simulink model "AmplitudeModulation"  (Simulink 7.5)
settings: Solver=ode45  StartTime=0.0  StopTime=5  RelTol=1e-3
settings Model: Creator=Terje B  LastModifiedBy=Terje B
settings DebuggingCC: SolverPrmCheckMsg=none

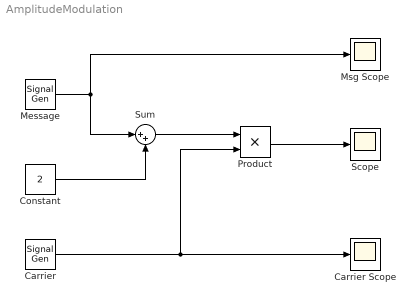
== system AmplitudeModulation ==
  Carrier : SignalGenerator  Frequency=10
  Carrier Scope : Scope
      settings: SaveName=ScopeData2
  Constant : Constant  Value=2  OutDataType=fixdt(1, 16)  OutScaling=2^0
  Message : SignalGenerator
  Msg Scope : Scope
  Product : Product  OutDataType=fixdt(1, 16)  OutScaling=2^0  SampleTime=.001  RndMeth=Zero
  Scope : Scope
  Sum : Sum  Inputs=|++  OutDataType=fixdt(1, 16)  OutScaling=2^0
  wires:
  Message/1 -> Sum/1, Msg Scope/1
  Constant/1 -> Sum/2
  Sum/1 -> Product/1
  Carrier/1 -> Product/2, Carrier Scope/1
  Product/1 -> Scope/1
